simulink library "xps_library"  (R2018a)
settings: Solver=ode45  StartTime=0.0  StopTime=10.0  RelTol=1e-3
undefined symbols (not defined in the file or in its folder): ip_name, lib_path
libraries: xbsIndex_r4 x2548, casper_library_flow_control x68, simulink x52, $bdroot x22, casper_library_misc x9
(part 7 of 30)

== system xps_library/DACs/red_pitaya_dac ==
  dac_reset_in : Inport
  dac_data_valid_in : Inport  Port=2
  dac0_data_i_in : Inport  Port=3
  dac1_data_q_in : Inport  Port=4
  convert_dac0_data_i_in : xbsIndex_r4/Convert  gui_display_data_type=Fixed-point  arith_type="Signed  (2's comp)"  n_bits=10  bin_pt=0  float_type=Single  exp_bits=8  fraction_bits=24  quantization=Truncate  overflow=Wrap  en=off  latency=0  pipeline=off  dbl_ovrd=off  block_type=convert
  convert_dac1_data_q_in1 : xbsIndex_r4/Convert  gui_display_data_type=Fixed-point  arith_type="Signed  (2's comp)"  n_bits=10  bin_pt=0  float_type=Single  exp_bits=8  fraction_bits=24  quantization=Truncate  overflow=Wrap  en=off  latency=0  pipeline=off  dbl_ovrd=off  block_type=convert
  convert_dac_data_valid_in : xbsIndex_r4/Convert  gui_display_data_type=Boolean  arith_type=Boolean  n_bits=16  bin_pt=14  float_type=Single  exp_bits=8  fraction_bits=24  quantization=Truncate  overflow=Wrap  en=off  latency=0  pipeline=off  dbl_ovrd=off  block_type=convert
  convert_dac_reset_in : xbsIndex_r4/Convert  gui_display_data_type=Boolean  arith_type=Boolean  n_bits=16  bin_pt=14  float_type=Single  exp_bits=8  fraction_bits=24  quantization=Truncate  overflow=Wrap  en=off  latency=0  pipeline=off  dbl_ovrd=off  block_type=convert
  xps_library_DACs_red_pitaya_dac_dac0_data_i_in : xbsIndex_r4/Gateway Out  inherit_from_input=off  hdl_port=on  rows=1  columns=1  UseAsDAC=off  DACChannel='1'  interface=None  automatic_assignment=on  address_offset=hex2dec('00')  intf_name=''  intf_description=''  timing_constraint=None  locs_specified=off  LOCs={}  io_standard={}  block_type=gatewayout
  xps_library_DACs_red_pitaya_dac_dac1_data_q_in : xbsIndex_r4/Gateway Out  inherit_from_input=off  hdl_port=on  rows=1  columns=1  UseAsDAC=off  DACChannel='1'  interface=None  automatic_assignment=on  address_offset=hex2dec('00')  intf_name=''  intf_description=''  timing_constraint=None  locs_specified=off  LOCs={}  io_standard={}  block_type=gatewayout
  xps_library_DACs_red_pitaya_dac_dac_data_valid_in : xbsIndex_r4/Gateway Out  inherit_from_input=off  hdl_port=on  rows=1  columns=1  UseAsDAC=off  DACChannel='1'  interface=None  automatic_assignment=on  address_offset=hex2dec('00')  intf_name=''  intf_description=''  timing_constraint=None  locs_specified=off  LOCs={}  io_standard={}  block_type=gatewayout
  xps_library_DACs_red_pitaya_dac_dac_reset_in : xbsIndex_r4/Gateway Out  inherit_from_input=off  hdl_port=on  rows=1  columns=1  UseAsDAC=off  DACChannel='1'  interface=None  automatic_assignment=on  address_offset=hex2dec('00')  intf_name=''  intf_description=''  timing_constraint=None  locs_specified=off  LOCs={}  io_standard={}  block_type=gatewayout
  wires:
  dac1_data_q_in/1 -> convert_dac1_data_q_in1/1
  convert_dac1_data_q_in1/1 -> xps_library_DACs_red_pitaya_dac_dac1_data_q_in/1
  convert_dac0_data_i_in/1 -> xps_library_DACs_red_pitaya_dac_dac0_data_i_in/1
  dac0_data_i_in/1 -> convert_dac0_data_i_in/1
  convert_dac_data_valid_in/1 -> xps_library_DACs_red_pitaya_dac_dac_data_valid_in/1
  dac_data_valid_in/1 -> convert_dac_data_valid_in/1
  convert_dac_reset_in/1 -> xps_library_DACs_red_pitaya_dac_dac_reset_in/1
  dac_reset_in/1 -> convert_dac_reset_in/1
